simulink subsystem "S2"  (R2024b)
settings: Solver=VariableStepAuto  StartTime=0.0  StopTime=10.0  RelTol=1e-3
undefined symbols (not defined in the file): C, CC, DPL1ph, h, Half, Ll, nb_cell, numberOfCell, P_AC, Rdc, ResistanceM, Roff, Ron, Rt4, SampleTime, simetran, Ts, Zm
libraries: fl_lib x39, nesl_utility x33, ee_lib x20, simulink x6
(part 1 of 2)
Description:
  | MMC station 2
settings Model: Creator=Kyle

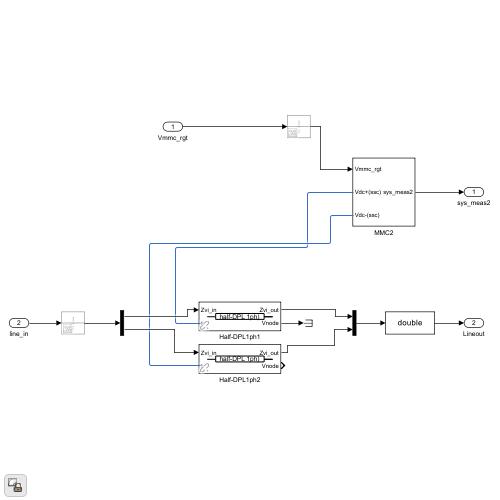
[thumbnail: Simulink's stored preview of the top-level diagram]
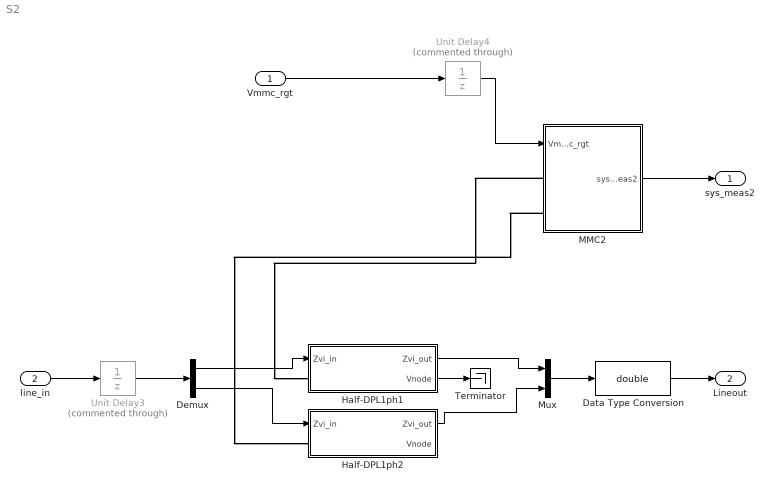
== system S2 ==
  Vmmc_rgt : Inport
  line_in : Inport  Port=2
  Data Type Conversion : DataTypeConversion  OutDataTypeStr=double  SaturateOnIntegerOverflow=off  RndMeth=Floor
  Demux : Demux  Outputs=2
  Half-DPL1ph1 : Subsystem  AncestorBlock=simetran/Half-DPL1ph  mask(Simscape 1-phase Distributed Parameters Line){Phases=1, Frequency=60, Resistance=0.015, Inductance=0.792e-3, Capacitance=14.4e-9, Length=300, Ts=Ts, cd=on}
      mask prompts: Phases "Number of phases N"; Frequency "Frequency used for R L C specification (Hz)"; Resistance "Resistance per unit length (Ohms/km)   [N*N matrix] or [R1 R0 R0m]"; Inductance "Inductance per unit length (H/km) [N*N matrix ] or [L1 L0 L0m]"; Capacitance "Capacitance per unit length (F/km) [N*N matrix] or [C1 C0 C0m]"; Length "Line length (km)"; Ts "Sample time (s)"; cd "Compensate for explicit external Unit Delay of propagation"
      mask help:
      | Implements a single-phase distributed parameter line (DPL) model.
      |
      | This DPL model allows the decoupling of computational tasks at each line ends.
      mask init:
      | % Get current block
      | currentBlock = gcb;
      | 
      | % Get electric variables
      | [Zm,R,v,Ti,to,Rt4,h,Zimp,Zmat,Yphase,ResistanceM] = ssc_dpl_cb(gcb,'variable_mask_maskinitialization', Phases, Frequency, Resistance, Inductance, Capacitance, Length);
      | % nphase=Phases;
      | % [Zm,R,v,Ti]=powericon('Distributed Parameter Line Model',nphase,Frequency,Resistance,Inductance,Capacitance);
      | %         %[Zmxx,Rmxx,Smodexx,Tixx] = blmodlin(nphase,Frequency,Resistance,Inductance,Capacitance);
      | %         %warning(w);
      | % 
      | % 
      | %         to = Length ./ v;
      | %         Rt4 = R * Length / 4;
      | %         h = (Zm - Rt4) ./ (Zm + Rt4);
      | %         Zimp = Zm + Rt4;
      | % 
      | %         % Calculate Zmat
      | %         Zmat = zeros(nphase);
      | %         for t = 1 : nphase
      | %             Zmat(t,t) = Zimp(t);
      | %         end
      | % 
      | %         % Calculate Y phase
      | %         Yphase=Ti*inv(Zmat)*(Ti');
      | % 
      | %         % Calculate R_x_0
      | %         ResistanceM = zeros(nphase);
      | %         for t = 1 : nphase
      | %             ResistanceM(t,t) = 1/(sum(Yphase(t,1:nphase)));
      | %         end
      | % 
      | %         % Calculate R_m_n
      | %         for t = 1 : nphase
      | %             for u = t+1: nphase
      | %                 ResistanceM(t,u) = -1/(Yphase(u,t));
      | %             end
      | %         end
      | V1_init=[0 zeros(1,Phases); 0.1 zeros(1,Phases)];
      | delay=floor(to/Ts);
      | if cd==1
      |     delay=delay-1;
      | end
      | if delay<1
      |     error('Line delay is less than 1 time step');
      | end
      | remd=rem(to,Ts)/Ts;
      mask TypeOptions Phases: 1 | 2 | 3 | 4 | 5 | 6 | 8 | 9 | 10 | 12
      mask Display:
      | plot(0,0,100,100,[20,20,80,80,90,80,80,20,20,10],[50,40,40,50,50,50,61,61,50,50])
      | disp('half-DPL 1ph)')
      | %disp(mess)
  Half-DPL1ph2 : Subsystem  AncestorBlock=simetran/Half-DPL1ph  mask(Simscape 1-phase Distributed Parameters Line){Phases=1, Frequency=60, Resistance=0.015, Inductance=0.792e-3, Capacitance=14.4e-9, Length=300, Ts=Ts, cd=on}
      mask prompts: Phases "Number of phases N"; Frequency "Frequency used for R L C specification (Hz)"; Resistance "Resistance per unit length (Ohms/km)   [N*N matrix] or [R1 R0 R0m]"; Inductance "Inductance per unit length (H/km) [N*N matrix ] or [L1 L0 L0m]"; Capacitance "Capacitance per unit length (F/km) [N*N matrix] or [C1 C0 C0m]"; Length "Line length (km)"; Ts "Sample time (s)"; cd "Compensate for explicit external Unit Delay of propagation"
      mask help:
      | Implements a single-phase distributed parameter line (DPL) model.
      |
      | This DPL model allows the decoupling of computational tasks at each line ends.
      mask init: same as S2/Half-DPL1ph1
      mask TypeOptions Phases: 1 | 2 | 3 | 4 | 5 | 6 | 8 | 9 | 10 | 12
      mask Display:
      | plot(0,0,100,100,[20,20,80,80,90,80,80,20,20,10],[50,40,40,50,50,50,61,61,50,50])
      | disp('half-DPL 1ph)')
      | %disp(mess)
  MMC2 : Subsystem
  Mux : Mux  Inputs=2
  Terminator : Terminator
  Unit Delay3 : UnitDelay  Commented=through  SampleTime=Ts  HasFrameUpgradeWarning=on
  Unit Delay4 : UnitDelay  Commented=through  SampleTime=Ts  HasFrameUpgradeWarning=on
  sys_meas2 : Outport
  Lineout : Outport  Port=2
  wires:
  Vmmc_rgt/1 -> Unit Delay4/1
  MMC2/1(sys_meas2) -> sys_meas2/1
  Unit Delay4/1 -> MMC2/1(Vmmc_rgt)
  Half-DPL1ph1/2(Vnode) -> Terminator/1
  Half-DPL1ph2/1(Zvi_out) -> Mux/2
  Mux/1 -> Data Type Conversion/1
  Half-DPL1ph1/1(Zvi_out) -> Mux/1
  line_in/1 -> Unit Delay3/1
  Demux/1 -> Half-DPL1ph1/1(Zvi_in)
  Demux/2 -> Half-DPL1ph2/1(Zvi_in)
  Unit Delay3/1 -> Demux/1
  Data Type Conversion/1 -> Lineout/1
  connections:
  MMC2/LConn1 -- Half-DPL1ph1/LConn1
  MMC2/LConn2 -- Half-DPL1ph2/LConn1

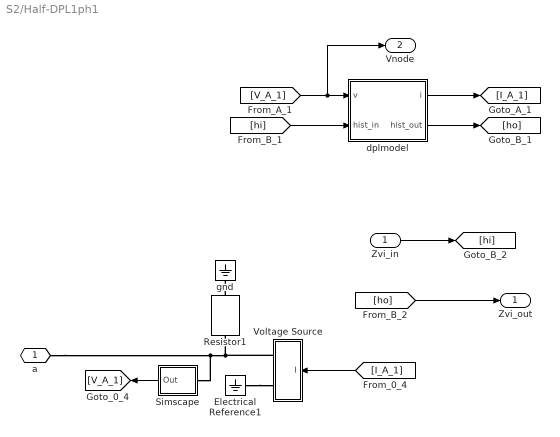
== system S2/Half-DPL1ph1 ==
  Zvi_in : Inport
  Electrical Reference1 : fl_lib/Electrical/Electrical Elements/Electrical Reference
  Resistor1 : ee_lib/Passive/Resistor  R=ResistanceM(1,1) Ohm  enable_R_tol=ee.enum.toleranceApplication.none  R_tol=5  tol_distribution=ee.enum.toleranceDistribution.uniform  nSigma=4  enable_operating_limits=ee.enum.enable.no  operating_limit_action=ee.enum.passive.reportOpLim.warn  power_rating=1 W  max_working_voltage=100 V  noise_mode=ee.enum.sources.noise.Disabled  Tdevice=25 degC  sample_time=1e-3 s  repeatability=ee.enum.ic.repeatability.notRepeatable  user_seed=0  auto_seed=3731015349  fault_action=simscape.enum.assert.action.none  t_fault=1 s  power_derating_T1=70 degC  power_derating_T2=155 degC  operating_temperature_range_vec=[-50, 150] degC  alpha=3.93e-3 1/K  Tmeas=25 degC  thermal_mass=100 J/K  temperature_specify=off  temperature_priority=High  temperature=298.15 K  temperature_nominal_specify=off  temperature_nominal_value=1  temperature_nominal_unit=K
  Simscape : Subsystem
      mask Display: disp('V')
  Voltage Source : Subsystem
  dplmodel : Subsystem
  gnd : fl_lib/Electrical/Electrical Elements/Electrical Reference
  a : PMIOPort  Side=Left
  Zvi_out : Outport  VectorParamsAs1DForOutWhenUnconnected=off
  Vnode : Outport  Port=2  VectorParamsAs1DForOutWhenUnconnected=off
  wires:
  [ho] -> Zvi_out/1
  dplmodel/1(i) -> [I_A_1]
  [V_A_1] -> Vnode/1, dplmodel/1(v)
  Zvi_in/1 -> [hi]
  [hi] -> dplmodel/2(hist_in)
  dplmodel/2(hist_out) -> [ho]
  Simscape/1(Out) -> [V_A_1]
  [I_A_1] -> Voltage Source/1(I)
  connections:
  a/RConn1 -- Simscape/LConn1 -- Voltage Source/RConn1 -- Resistor1/RConn1
  Resistor1/LConn1 -- gnd/LConn1
  Electrical Reference1/LConn1 -- Voltage Source/RConn2

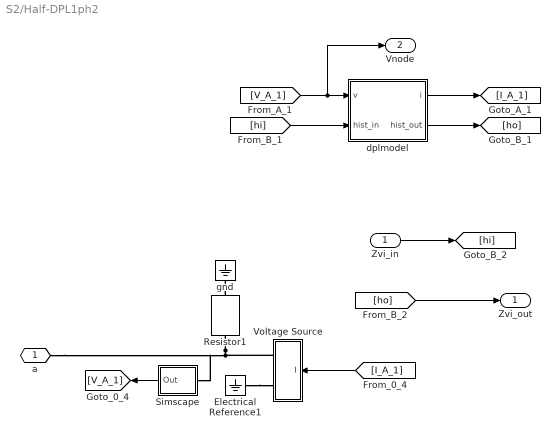
== system S2/Half-DPL1ph2 ==
  Zvi_in : Inport
  Electrical Reference1 : fl_lib/Electrical/Electrical Elements/Electrical Reference
  Resistor1 : ee_lib/Passive/Resistor  R=ResistanceM(1,1) Ohm  enable_R_tol=ee.enum.toleranceApplication.none  R_tol=5  tol_distribution=ee.enum.toleranceDistribution.uniform  nSigma=4  enable_operating_limits=ee.enum.enable.no  operating_limit_action=ee.enum.passive.reportOpLim.warn  power_rating=1 W  max_working_voltage=100 V  noise_mode=ee.enum.sources.noise.Disabled  Tdevice=25 degC  sample_time=1e-3 s  repeatability=ee.enum.ic.repeatability.notRepeatable  user_seed=0  auto_seed=362649195  fault_action=simscape.enum.assert.action.none  t_fault=1 s  power_derating_T1=70 degC  power_derating_T2=155 degC  operating_temperature_range_vec=[-50, 150] degC  alpha=3.93e-3 1/K  Tmeas=25 degC  thermal_mass=100 J/K  temperature_specify=off  temperature_priority=High  temperature=298.15 K  temperature_nominal_specify=off  temperature_nominal_value=1  temperature_nominal_unit=K
  Simscape : Subsystem
      mask Display: disp('V')
  Voltage Source : Subsystem
  dplmodel : Subsystem
  gnd : fl_lib/Electrical/Electrical Elements/Electrical Reference
  a : PMIOPort  Side=Left
  Zvi_out : Outport  VectorParamsAs1DForOutWhenUnconnected=off
  Vnode : Outport  Port=2  VectorParamsAs1DForOutWhenUnconnected=off
  wires:
  [I_A_1] -> Voltage Source/1(I)
  Simscape/1(Out) -> [V_A_1]
  dplmodel/2(hist_out) -> [ho]
  [hi] -> dplmodel/2(hist_in)
  Zvi_in/1 -> [hi]
  [V_A_1] -> dplmodel/1(v), Vnode/1
  dplmodel/1(i) -> [I_A_1]
  [ho] -> Zvi_out/1
  connections:
  Electrical Reference1/LConn1 -- Voltage Source/RConn2
  Resistor1/LConn1 -- gnd/LConn1
  Resistor1/RConn1 -- Voltage Source/RConn1 -- Simscape/LConn1 -- a/RConn1

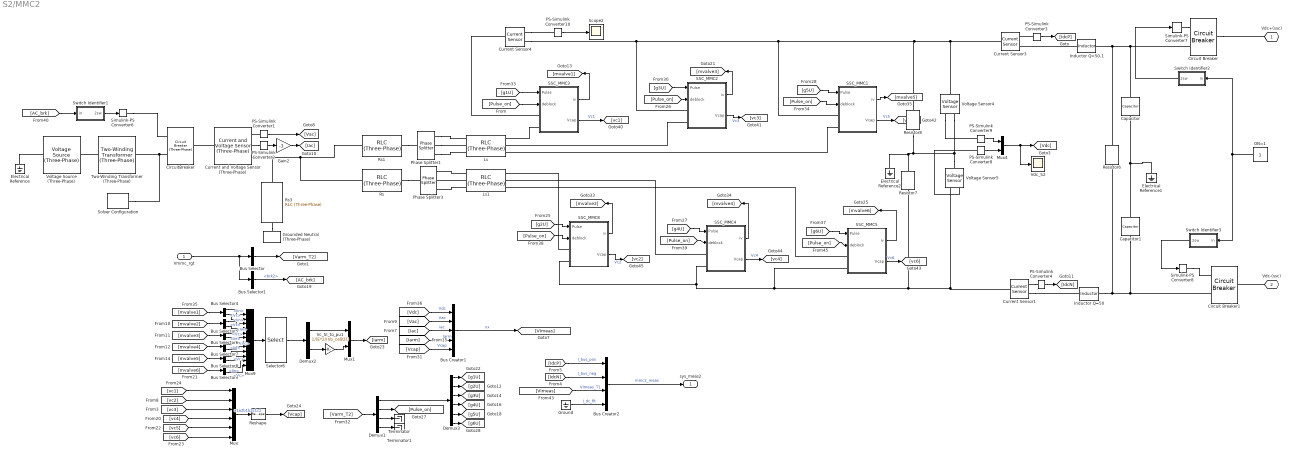
== system S2/MMC2 ==
  Vmmc_rgt : Inport
  " Switch Identifier1" : Subsystem  mask{bn=brk1, bns=brk1, rsw=on}
      mask prompts: bn "Switch block name (no ' ')"; bns "saved blockname"; rsw "Reverse switch logic"
      mask DialogControl Control2 Prompt: Note: Simscape electric breaker in open (OFF) when gate=1)
      mask DialogControl Control3 Prompt: Note: by using revert logic, it becomes like SPS breaker
  " Switch Identifier2" : Subsystem  mask{bn=brk1, bns=brk1, rsw=on}
      mask prompts: bn "Switch block name (no ' ')"; bns "saved blockname"; rsw "Reverse switch logic"
      mask DialogControl Control2 Prompt: Note: Simscape electric breaker in open (OFF) when gate=1)
      mask DialogControl Control3 Prompt: Note: by using revert logic, it becomes like SPS breaker
  " Switch Identifier3" : Subsystem  mask{bn=brk1, bns=brk1, rsw=on}
      mask prompts: bn "Switch block name (no ' ')"; bns "saved blockname"; rsw "Reverse switch logic"
      mask DialogControl Control2 Prompt: Note: Simscape electric breaker in open (OFF) when gate=1)
      mask DialogControl Control3 Prompt: Note: by using revert logic, it becomes like SPS breaker
  Bus Creator1 : BusCreator  Inputs=5
  Bus Creator2 : BusCreator  Inputs=4  OutDataTypeStr=Bus: mmc2_meas  NonVirtualBus=on
  Bus Selector : BusSelector  OutputSignals=pulse,dblk_rgt,para  OutputAsBus=on
  Bus Selector1 : BusSelector  OutputSignals=brk2
  Bus Selector{4..9} (6 alike) : BusSelector  OutputSignals=Iin,Vc
  Capacitor : ee_lib/Passive/Capacitor  cap_option=ee.enum.passive.capacitor.capOption.const  c=2.5e-6 F  Cvec=[1e-05, 1e-06] F  Vvec=[0, 10] V  CV_table_symmetry=ee.enum.passive.capacitor.tableSymmetry.yes  f_vec=[1, 10] kHz  DFext_vec=[.8, 1.2]  enable_C_tol=ee.enum.toleranceApplication.none  averaging_period=0 s  C_tol=5  tol_distribution=ee.enum.toleranceDistribution.uniform  nSigma=4  r=0 Ohm  g=0 1/Ohm  enable_operating_limits=ee.enum.enable.no  operating_limit_action=ee.enum.passive.reportOpLim.warn  max_working_voltage_range=[-25, 25] V  power_rating=1 W  maxTemperature=85 degC  thermalEnable=false  thermalMass=1 J/K  fault_action=simscape.enum.assert.action.none  t_fault=1 s  i_specify=off  i_priority=None  i=0 A  i_nominal_specify=off  i_nominal_value=1  i_nominal_unit=A  v_specify=off  v_priority=None  v=0 V  v_nominal_specify=off  v_nominal_value=1  v_nominal_unit=V  vc_specify=off  vc_priority=High  vc=0 V  vc_nominal_specify=off  vc_nominal_value=1  vc_nominal_unit=V  T_specify=off  T_priority=None  T=298.15 K  T_nominal_specify=off  T_nominal_value=1  T_nominal_unit=K
  Capacitor1 : ee_lib/Passive/Capacitor  cap_option=ee.enum.passive.capacitor.capOption.const  c=2.5e-6 F  Cvec=[1e-05, 1e-06] F  Vvec=[0, 10] V  CV_table_symmetry=ee.enum.passive.capacitor.tableSymmetry.yes  f_vec=[1, 10] kHz  DFext_vec=[.8, 1.2]  enable_C_tol=ee.enum.toleranceApplication.none  averaging_period=0 s  C_tol=5  tol_distribution=ee.enum.toleranceDistribution.uniform  nSigma=4  r=0 Ohm  g=0 1/Ohm  enable_operating_limits=ee.enum.enable.no  operating_limit_action=ee.enum.passive.reportOpLim.warn  max_working_voltage_range=[-25, 25] V  power_rating=1 W  maxTemperature=85 degC  thermalEnable=false  thermalMass=1 J/K  fault_action=simscape.enum.assert.action.none  t_fault=1 s  i_specify=off  i_priority=None  i=0 A  i_nominal_specify=off  i_nominal_value=1  i_nominal_unit=A  v_specify=off  v_priority=None  v=0 V  v_nominal_specify=off  v_nominal_value=1  v_nominal_unit=V  vc_specify=off  vc_priority=High  vc=0 V  vc_nominal_specify=off  vc_nominal_value=1  vc_nominal_unit=V  T_specify=off  T_priority=None  T=298.15 K  T_nominal_specify=off  T_nominal_value=1  T_nominal_unit=K
  Circuit Breaker : ee_lib/Switches & Breakers/Circuit Breaker  R_closed=0.001 Ohm  G_open=1e-6 1/Ohm  threshold=0.5 V  breaker_behavior=ee.enum.switches.breakerBehavior.zeroCrossingEnable
      settings: InternalSimscapePortConfiguration="{\"Bottom\":[],\"Left\":[{\"id\":\"vT\",\"label\":\"vT\",\"type\":\"input\"},{\"id\":\"p1\",\"label\":\"\",\"type\":\"foundation.electrical.electrical\"}],\"Right\":[{\"id\":\"p2\",\"label\":\"\",\"type\":\"foundation.electrical.electrical\"}],\"Top\":[]}"
  Circuit Breaker1 : ee_lib/Switches & Breakers/Circuit Breaker  R_closed=0.001 Ohm  G_open=1e-6 1/Ohm  threshold=0.5 V  breaker_behavior=ee.enum.switches.breakerBehavior.zeroCrossingEnable
      settings: InternalSimscapePortConfiguration="{\"Bottom\":[],\"Left\":[{\"id\":\"vT\",\"label\":\"vT\",\"type\":\"input\"},{\"id\":\"p1\",\"label\":\"\",\"type\":\"foundation.electrical.electrical\"}],\"Right\":[{\"id\":\"p2\",\"label\":\"\",\"type\":\"foundation.electrical.electrical\"}],\"Top\":[]}"
  CircuitBreaker : ee_lib/Switches & Breakers/Circuit Breaker (Three-Phase)  R_closed=0.001 Ohm  G_open=1/1000 1/Ohm  threshold=0.5 V  breaker_behavior=ee.enum.switches.breakerBehavior.zeroCrossingEnable
      settings: InternalSimscapePortConfiguration="{\"Bottom\":[],\"Left\":[{\"id\":\"vT\",\"label\":\"vT\",\"type\":\"input\"},{\"id\":\"N1\",\"label\":\"~1\",\"type\":\"foundation.electrical.three_phase\"}],\"Right\":[{\"id\":\"N2\",\"label\":\"~2\",\"type\":\"foundation.electrical.three_phase\"}],\"Top\":[]}"
  Current Sensor1 : fl_lib/Electrical/Electrical Sensors/Current Sensor
  Current Sensor3 : fl_lib/Electrical/Electrical Sensors/Current Sensor
  Current Sensor4 : fl_lib/Electrical/Electrical Sensors/Current Sensor
  Current and Voltage Sensor (Three-Phase) : ee_lib/Sensors & Transducers/Current and Voltage Sensor (Three-Phase)  vMeasurementType=ee.enum.vmeasurement.lg  outputUnit=ee.enum.unit.si  SRated=100e6 A*V  VRated=24e3 V  I_specify=off  I_priority=None  I=[0, 0, 0] A  I_nominal_specify=off  I_nominal_value=1  I_nominal_unit=A  V_specify=off  V_priority=None  V=[0, 0, 0] V  V_nominal_specify=off  V_nominal_value=1  V_nominal_unit=V
      settings: InternalSimscapePortConfiguration="{\"Bottom\":[],\"Left\":[{\"id\":\"N1\",\"label\":\"~1\",\"type\":\"foundation.electrical.three_phase\"}],\"Right\":[{\"id\":\"V_output\",\"label\":\"V\",\"type\":\"output\"},{\"id\":\"I_output\",\"label\":\"I\",\"type\":\"output\"},{\"id\":\"N2\",\"label\":\"~2\",\"type\":\"foundation.electrical.three_phase\"}],\"Top\":[]}"
  Demux1 : Demux  Outputs=[numberOfCell*6 1 5 1]
  Demux2 : Demux  Outputs=[6 6]
  Demux3 : Demux  Outputs=ones(6,1)*numberOfCell
  Electrical Reference : fl_lib/Electrical/Electrical Elements/Electrical Reference
  Electrical Reference1 : fl_lib/Electrical/Electrical Elements/Electrical Reference
  Electrical Reference2 : fl_lib/Electrical/Electrical Elements/Electrical Reference
  Gain2 : Gain  Gain=-1
  Ground : Ground
  Grounded Neutral (Three-Phase) : ee_lib/Connectors & References/Grounded Neutral (Three-Phase)
  Inductor Q=50 : ee_lib/Passive/Inductor  l=10e-3 H  enable_L_tol=ee.enum.toleranceApplication.none  L_tol=20  tol_distribution=ee.enum.toleranceDistribution.uniform  nSigma=4  r=2*pi*50/50*10e-3 Ohm  g=1e-9 1/Ohm  enable_operating_limits=ee.enum.enable.no  operating_limit_action=ee.enum.passive.reportOpLim.warn  max_working_current=1 A  power_rating=1 W  fault_action=simscape.enum.assert.action.none  t_fault=1 s  i_L_specify=off  i_L_priority=High  i_L=0 A  i_L_nominal_specify=off  i_L_nominal_value=1  i_L_nominal_unit=A
  Inductor Q=50.1 : ee_lib/Passive/Inductor  l=10e-3 H  enable_L_tol=ee.enum.toleranceApplication.none  L_tol=20  tol_distribution=ee.enum.toleranceDistribution.uniform  nSigma=4  r=2*pi*50/50*10e-3 Ohm  g=1e-9 1/Ohm  enable_operating_limits=ee.enum.enable.no  operating_limit_action=ee.enum.passive.reportOpLim.warn  max_working_current=1 A  power_rating=1 W  fault_action=simscape.enum.assert.action.none  t_fault=1 s  i_L_specify=off  i_L_priority=High  i_L=0 A  i_L_nominal_specify=off  i_L_nominal_value=1  i_L_nominal_unit=A
  Ls : ee_lib/Passive/RLC Assemblies/RLC (Three-Phase)  port_option=ee.enum.threePhasePort.expanded  component_structure=ee.enum.rlc.structure.ParallelRL  R=Ll*2*pi*10000 Ohm  L=Ll H  C=1e-6 F  R_parasitic=0 Ohm  G_parasitic=0 1/Ohm  IL_specify=off  IL_priority=High  IL=[0, 0, 0] A  IL_nominal_specify=off  IL_nominal_value=1  IL_nominal_unit=A  VC_specify=off  VC_priority=High  VC=[0, 0, 0] V  VC_nominal_specify=off  VC_nominal_value=1  VC_nominal_unit=V
      settings: InternalSimscapePortConfiguration="{\"Bottom\":[],\"Left\":[{\"id\":\"a1\",\"label\":\"a1\",\"type\":\"foundation.electrical.electrical\"},{\"id\":\"b1\",\"label\":\"b1\",\"type\":\"foundation.electrical.electrical\"},{\"id\":\"c1\",\"label\":\"c1\",\"type\":\"foundation.electrical.electrical\"}],\"Right\":[{\"id\":\"a2\",\"label\":\"a2\",\"type\":\"foundation.electrical.electrical\"},{\"id\":\"b2\",\"label\":\"b2\",\"type\":\"foundation.electrical.electrical\"},{\"id\":\"c2\",\"label\":\"c2\",\"type\":\"foundation.electrical.electrical\"}],\"Top\":[]}"
  Ls1 : ee_lib/Passive/RLC Assemblies/RLC (Three-Phase)  port_option=ee.enum.threePhasePort.expanded  component_structure=ee.enum.rlc.structure.ParallelRL  R=Ll*2*pi*10000 Ohm  L=Ll H  C=1e-6 F  R_parasitic=0 Ohm  G_parasitic=0 1/Ohm  IL_specify=off  IL_priority=High  IL=[0, 0, 0] A  IL_nominal_specify=off  IL_nominal_value=1  IL_nominal_unit=A  VC_specify=off  VC_priority=High  VC=[0, 0, 0] V  VC_nominal_specify=off  VC_nominal_value=1  VC_nominal_unit=V
      settings: InternalSimscapePortConfiguration="{\"Bottom\":[],\"Left\":[{\"id\":\"a1\",\"label\":\"a1\",\"type\":\"foundation.electrical.electrical\"},{\"id\":\"b1\",\"label\":\"b1\",\"type\":\"foundation.electrical.electrical\"},{\"id\":\"c1\",\"label\":\"c1\",\"type\":\"foundation.electrical.electrical\"}],\"Right\":[{\"id\":\"a2\",\"label\":\"a2\",\"type\":\"foundation.electrical.electrical\"},{\"id\":\"b2\",\"label\":\"b2\",\"type\":\"foundation.electrical.electrical\"},{\"id\":\"c2\",\"label\":\"c2\",\"type\":\"foundation.electrical.electrical\"}],\"Top\":[]}"
  Mux : Mux  Inputs=ones(6,1)*numberOfCell
  Mux1 : Mux  Inputs=2
  Mux4 : Mux  Inputs=2
  Mux9 : Mux  Inputs=12
  ON=1 : Constant
  PS-Simulink Converter{1..4,8..10} (7 alike) : nesl_utility/PS-Simulink Converter  PhysicalDomain=network_engine_domain  SubClassName=ps_output  LeftPortType=input  RightPortType=output  PseudoPeriodic=off  Frequencies=[]  VectorFormat=inherit  Unit=inherit  AffineConversion=off
  Phase Splitter1 : ee_lib/Connectors & References/Phase Splitter
  Phase Splitter3 : ee_lib/Connectors & References/Phase Splitter
  Reshape : Reshape
  Resistor6 : fl_lib/Electrical/Electrical Elements/Resistor  R=1000000 Ohm  i_specify=off  i_priority=None  i=0 A  i_nominal_specify=off  i_nominal_value=1  i_nominal_unit=A  v_specify=off  v_priority=None  v=0 V  v_nominal_specify=off  v_nominal_value=1  v_nominal_unit=V
  Resistor7 : fl_lib/Electrical/Electrical Elements/Resistor  R=Rdc Ohm  i_specify=off  i_priority=None  i=0 A  i_nominal_specify=off  i_nominal_value=1  i_nominal_unit=A  v_specify=off  v_priority=None  v=0 V  v_nominal_specify=off  v_nominal_value=1  v_nominal_unit=V
  Resistor8 : fl_lib/Electrical/Electrical Elements/Resistor  R=Rdc Ohm  i_specify=off  i_priority=None  i=0 A  i_nominal_specify=off  i_nominal_value=1  i_nominal_unit=A  v_specify=off  v_priority=None  v=0 V  v_nominal_specify=off  v_nominal_value=1  v_nominal_unit=V
  Rs : ee_lib/Passive/RLC Assemblies/RLC (Three-Phase)  port_option=ee.enum.threePhasePort.composite  component_structure=ee.enum.rlc.structure.R  R=0.0001 Ohm  L=Ll H  C=1e-6 F  R_parasitic=0 Ohm  G_parasitic=0 1/Ohm  IL_specify=off  IL_priority=High  IL=[0, 0, 0] A  IL_nominal_specify=off  IL_nominal_value=1  IL_nominal_unit=A  VC_specify=off  VC_priority=High  VC=[0, 0, 0] V  VC_nominal_specify=off  VC_nominal_value=1  VC_nominal_unit=V
      settings: InternalSimscapePortConfiguration="{\"Bottom\":[],\"Left\":[{\"id\":\"N1\",\"label\":\"~1\",\"type\":\"foundation.electrical.three_phase\"}],\"Right\":[{\"id\":\"N2\",\"label\":\"~2\",\"type\":\"foundation.electrical.three_phase\"}],\"Top\":[]}"
  Rs1 : ee_lib/Passive/RLC Assemblies/RLC (Three-Phase)  port_option=ee.enum.threePhasePort.composite  component_structure=ee.enum.rlc.structure.R  R=0.0001 Ohm  L=Ll H  C=1e-6 F  R_parasitic=0 Ohm  G_parasitic=0 1/Ohm  IL_specify=off  IL_priority=High  IL=[0, 0, 0] A  IL_nominal_specify=off  IL_nominal_value=1  IL_nominal_unit=A  VC_specify=off  VC_priority=High  VC=[0, 0, 0] V  VC_nominal_specify=off  VC_nominal_value=1  VC_nominal_unit=V
      settings: InternalSimscapePortConfiguration="{\"Bottom\":[],\"Left\":[{\"id\":\"N1\",\"label\":\"~1\",\"type\":\"foundation.electrical.three_phase\"}],\"Right\":[{\"id\":\"N2\",\"label\":\"~2\",\"type\":\"foundation.electrical.three_phase\"}],\"Top\":[]}"
  Rs3 : ee_lib/Passive/RLC Assemblies/RLC (Three-Phase)  port_option=ee.enum.threePhasePort.composite  component_structure=ee.enum.rlc.structure.R  R=1e6 Ohm  L=Ll H  C=1e-6 F  R_parasitic=0 Ohm  G_parasitic=0 1/Ohm  IL_specify=off  IL_priority=High  IL=[0, 0, 0] A  IL_nominal_specify=off  IL_nominal_value=1  IL_nominal_unit=A  VC_specify=off  VC_priority=High  VC=[0, 0, 0] V  VC_nominal_specify=off  VC_nominal_value=1  VC_nominal_unit=V
      settings: InternalSimscapePortConfiguration="{\"Bottom\":[],\"Left\":[{\"id\":\"N1\",\"label\":\"~1\",\"type\":\"foundation.electrical.three_phase\"}],\"Right\":[{\"id\":\"N2\",\"label\":\"~2\",\"type\":\"foundation.electrical.three_phase\"}],\"Top\":[]}"
  SSC_MMC1 : Subsystem  mask(SimScape MMC module (half-bridge)){nbc=200, ron=Ron, roff=Roff, cc=CC, Ts=Ts, rf=on, dts=on}
      mask prompts: nbc "Number of cell"; ron "IGBT Ron (Ohms)"; roff "IGBT Roff (Ohms)"; cc "Cell capacitance (F)"; Ts "Sample Time (s)"; rf "Non-infinite Roff"; dts "Disabled time stamping"
      mask help: This model implements an half-bridge MMC module with full nodal solution, i.e. there is no delay between the MMC and then main solver solution and the MMC module is seen as a discrete Thevenin equivalent to the main Simscape solver.
      mask init:
      | for k=1:4
      |     switch k
      |          case 1
      |               R1=roff; R2=roff;
      |               A(k)=0; B(k)=0; C(k)=0; D(k)=R2;
      |          case 2
      |               R1=ron; R2=roff;
      |               A(k)=0; B(k)=1/cc; C(k)=1; D(k)=R1;
      |          case 3
      |               R1=roff; R2=ron;
      |               A(k)=0; B(k)=0; C(k)=0; D(k)=R2;
      |          case 4
      |              R1=ron; R2=ron;
      |              A(k)=0; B(k)=0; C(k)=0; D(k)=R2; %incorrect but not supposed to happen
      |     end
      |     if isequal(get_param(gcb,'rf'),'on')
      |      rr=(1+R2/R1);
      |      A(k)=-1/R1/cc/rr;
      |      B(k)=R2/R1/cc/rr;
      |      C(k)=R2/R1/rr;
      |      D(k)=R2/rr;
      |     end
      |          
      |        %% choose here if you want trapeze or backward Euler (more stable) 
      |         if 1==0 % trap
      |             Ad(k) = (1-Ts/2*A(k))\(1+Ts/2*A(k));         %SS discretize
      |             Bd1(k) = (1-Ts/2*A(k))\(Ts/2*B(k));    %SS discretize
      |             Bd2(k) = (1-Ts/2*A(k))\(Ts/2*B(k));    %SS discretize
      |         else % BE
      |             Ad(k) = 1/(1-Ts*A(k));         %SS discretize
      |             Bd2(k) = Ts*B(k)/(1-Ts*A(k));    %SS discretize
      |             Bd1(k) =0;
      |         end
      |         Z(k)=C(k)'.*Bd2(k) + D(k);
      | end
      | 
      | 
      | dtsval=1; %must be = 1
      mask Display: disp('MMC arm')
  SSC_MMC2 : Subsystem  mask(SimScape MMC module (half-bridge)){nbc=200, ron=Ron, roff=Roff, cc=CC, Ts=Ts, rf=on, dts=on}
      mask prompts: nbc "Number of cell"; ron "IGBT Ron (Ohms)"; roff "IGBT Roff (Ohms)"; cc "Cell capacitance (F)"; Ts "Sample Time (s)"; rf "Non-infinite Roff"; dts "Disabled time stamping"
      mask help: This model implements an half-bridge MMC module with full nodal solution, i.e. there is no delay between the MMC and then main solver solution and the MMC module is seen as a discrete Thevenin equivalent to the main Simscape solver.
      mask init: same as S2/MMC2/SSC_MMC1
      mask Display: disp('MMC arm')
  SSC_MMC3 : Subsystem  mask(SimScape MMC module (half-bridge)){nbc=200, ron=Ron, roff=Roff, cc=CC, Ts=Ts, rf=on, dts=on}
      mask prompts: nbc "Number of cell"; ron "IGBT Ron (Ohms)"; roff "IGBT Roff (Ohms)"; cc "Cell capacitance (F)"; Ts "Sample Time (s)"; rf "Non-infinite Roff"; dts "Disabled time stamping"
      mask help: This model implements an half-bridge MMC module with full nodal solution, i.e. there is no delay between the MMC and then main solver solution and the MMC module is seen as a discrete Thevenin equivalent to the main Simscape solver.
      mask init: same as S2/MMC2/SSC_MMC1
      mask Display: disp('MMC arm')
  SSC_MMC4 : Subsystem  mask(SimScape MMC module (half-bridge)){nbc=200, ron=Ron, roff=Roff, cc=CC, Ts=Ts, rf=on, dts=on}
      mask prompts: nbc "Number of cell"; ron "IGBT Ron (Ohms)"; roff "IGBT Roff (Ohms)"; cc "Cell capacitance (F)"; Ts "Sample Time (s)"; rf "Non-infinite Roff"; dts "Disabled time stamping"
      mask help: This model implements an half-bridge MMC module with full nodal solution, i.e. there is no delay between the MMC and then main solver solution and the MMC module is seen as a discrete Thevenin equivalent to the main Simscape solver.
      mask init: same as S2/MMC2/SSC_MMC1
      mask Display: disp('MMC arm')
  SSC_MMC5 : Subsystem  mask(SimScape MMC module (half-bridge)){nbc=200, ron=Ron, roff=Roff, cc=CC, Ts=Ts, rf=on, dts=on}
      mask prompts: nbc "Number of cell"; ron "IGBT Ron (Ohms)"; roff "IGBT Roff (Ohms)"; cc "Cell capacitance (F)"; Ts "Sample Time (s)"; rf "Non-infinite Roff"; dts "Disabled time stamping"
      mask help: This model implements an half-bridge MMC module with full nodal solution, i.e. there is no delay between the MMC and then main solver solution and the MMC module is seen as a discrete Thevenin equivalent to the main Simscape solver.
      mask init: same as S2/MMC2/SSC_MMC1
      mask Display: disp('MMC arm')
  SSC_MMC8 : Subsystem  mask(SimScape MMC module (half-bridge)){nbc=200, ron=Ron, roff=Roff, cc=CC, Ts=Ts, rf=on, dts=on}
      mask prompts: nbc "Number of cell"; ron "IGBT Ron (Ohms)"; roff "IGBT Roff (Ohms)"; cc "Cell capacitance (F)"; Ts "Sample Time (s)"; rf "Non-infinite Roff"; dts "Disabled time stamping"
      mask help: This model implements an half-bridge MMC module with full nodal solution, i.e. there is no delay between the MMC and then main solver solution and the MMC module is seen as a discrete Thevenin equivalent to the main Simscape solver.
      mask init: same as S2/MMC2/SSC_MMC1
      mask Display: disp('MMC arm')
  Scope2 : Scope
  Selector6 : Selector  InputPortWidth=12  IndexOptions=Index vector (dialog)  Indices=[1:2:12,2:2:12]  OutputSizes=1
  Simulink-PS Converter6 : nesl_utility/Simulink-PS Converter  PhysicalDomain=network_engine_domain  SubClassName=ps_input  LeftPortType=input  RightPortType=output  PseudoPeriodic=off  Frequencies=[]  NoiseDistribution=none  NoiseParameters=[]  Unit=1  AffineConversion=off  FilteringAndDerivatives=provide  SimscapeFilterOrder=1  InputFilterTimeConstant=0.001  UdotUserProvided=0
  Simulink-PS Converter7 : nesl_utility/Simulink-PS Converter  PhysicalDomain=network_engine_domain  SubClassName=ps_input  LeftPortType=input  RightPortType=output  PseudoPeriodic=off  Frequencies=[]  NoiseDistribution=none  NoiseParameters=[]  Unit=1  AffineConversion=off  FilteringAndDerivatives=provide  SimscapeFilterOrder=1  InputFilterTimeConstant=0.001  UdotUserProvided=0
  Simulink-PS Converter8 : nesl_utility/Simulink-PS Converter  PhysicalDomain=network_engine_domain  SubClassName=ps_input  LeftPortType=input  RightPortType=output  PseudoPeriodic=off  Frequencies=[]  NoiseDistribution=none  NoiseParameters=[]  Unit=1  AffineConversion=off  FilteringAndDerivatives=provide  SimscapeFilterOrder=1  InputFilterTimeConstant=0.001  UdotUserProvided=0
  Solver Configuration : nesl_utility/Solver Configuration  PhysicalDomain=network_engine_domain  SubClassName=solver  LeftPortType=input  RightPortType=generic  Tones=[]  Harmonics=[]  SimulateNoise=off  Profile=off  UseLocalSampling=off  EnableSwitchedLinearOptims=on  FrequencyDomain=off  UseCCode=off  RelTol=0.001  AbsTol=0.001  MinStep=1e-09  ToWorkspace=off  RevertToSquareIcSolve=off  NumHomotopyIterations=100  PhasorMode=off  PhasorModeNumHarmonics=1  ConsistencySolver=NEWTON_XTOL_AFTER_FTOL  IndexReductionMethod=None  DoDC=off  ResidualTolerance=1e-09  ConsistencyTolSource=GLOBAL  ConsistencyAbsTol=0.001  ConsistencyRelTol=0.001  ConsistencyTolFactor=0.001  UseLocalSolver=on  LocalSolverChoice=NE_TRAPEZOIDAL_ADVANCER  ResolveIndetEquations=off  FunctionEvalNumThread=1  LocalSolverSampleTime=Ts  DoFixedCost=on  MaxNonlinIter=1  MaxModeIter=2  ComputeImpulses=off  ImpulseIterations=2  LinearAlgebra=auto  LinearAlgebraNumThread=0  EquationFormulation=NE_TIME_EF  DelaysMemoryBudget=1024  AutomaticFiltering=off  FilteringTimeConstant=0.001  PartitionStorageMethod=AS_NEEDED  PartitionMemoryBudget=1024  PartitionMethod=ROBUST  MultibodyUseLocalSolver=off  MultibodyLocalSolverChoice=ODE1  MultibodyLocalSolverSampleTime=0.001
  Terminator : Terminator
  Terminator1 : Terminator
  Two-Winding Transformer (Three-Phase) : ee_lib/Passive/Transformers/Two-Winding Transformer (Three-Phase)  SRated=S_Xfo A*V  FRated=freq_right Hz  Winding1Connection=ee.enum.windingconnection.Yg  VRated1="V_AC_prim   V"  Winding2Connection=ee.enum.windingconnection.Y  VRated2=V_AC_sec V  CoreType=ee.enum.coretype.fivelimb  pu_Rw1=0.0025  pu_Rw2=0.0025  leakage_reactance_option=ee.enum.transformer_leakage.include  pu_Xl1=0.05  pu_Xl2=0.05  magnetizing_resistance_option=ee.enum.transformer_magnetizingResistance.include  pu_Rm=167  magnetizing_reactance_option=ee.enum.transformer_magnetizingReactance.include  saturation_option=ee.enum.transformer_saturation.exclude  pu_Xm=167  current_data=[0, .002, 1, 2]  magnetic_flux_data=[0, 1.2, 1.5, 1.51]  pu_X0=0.5  i1_specify=off  i1_priority=None  i1=[0, 0, 0] A  i1_nominal_specify=off  i1_nominal_value=1  i1_nominal_unit=A  i2_specify=off  i2_priority=None  i2=[0, 0, 0] A  i2_nominal_specify=off  i2_nominal_value=1  i2_nominal_unit=A  phi_specify=off  phi_priority=None  phi=[0, 0, 0]  phi_nominal_specify=off  phi_nominal_value=1  phi_nominal_unit=1  power_dissipated_specify=off  power_dissipated_priority=None  power_dissipated=0 W  power_dissipated_nominal_specify=off  power_dissipated_nominal_value=1  power_dissipated_nominal_unit=W
      settings: InternalSimscapePortConfiguration="{\"Bottom\":[],\"Left\":[{\"id\":\"N1\",\"label\":\"~1\",\"type\":\"foundation.electrical.three_phase\"}],\"Right\":[{\"id\":\"N2\",\"label\":\"~2\",\"type\":\"foundation.electrical.three_phase\"}],\"Top\":[]}"
  Vc_SI_to_pu1 : Gain  Gain=1/(E*2/(nb_cell/2))  SampleTime=Ts
  Vdc_S2 : Scope
  Voltage Source (Three-Phase) : ee_lib/Sources/Voltage Source (Three-Phase)  vline_rms=V_AC_prim V  shift=0 deg  freq=freq_right Hz  impedance_option=1  SShortCircuit=P_AC*20 A*V  XR=20  R=0.01 Ohm  L=3.97e-4 H  harmonic_option=0  harmonic_orders=[5, 7, 11, 13]  harmonic_ratios=[.1, .1, .1, .1]  G_parasitic=0 1/Ohm  I_specify=off  I_priority=None  I=[0, 0, 0] A  I_nominal_specify=off  I_nominal_value=1  I_nominal_unit=A
  Voltage Sensor4 : fl_lib/Electrical/Electrical Sensors/Voltage Sensor
  Voltage Sensor5 : fl_lib/Electrical/Electrical Sensors/Voltage Sensor
  Vdc+(ssc) : PMIOPort  Tag=PMCPort  Side=Left
  Vdc-(ssc) : PMIOPort  Tag=PMCPort  Port=2  Side=Left
  sys_meas2 : Outport  VectorParamsAs1DForOutWhenUnconnected=off
  wires:
  [g3U] -> SSC_MMC2/1(Pulse)
  [g1U] -> SSC_MMC3/1(Pulse)
  [Pulse_on] -> SSC_MMC3/2(deblock)
  ON=1/1 -> " Switch Identifier3"/1(in), " Switch Identifier2"/1(in)
  PS-Simulink Converter9/1 -> Mux4/1
  SSC_MMC5/2(Vcap) -> [vc6]  "Vc6"
  SSC_MMC5/1(iv) -> [mvalve6]
  SSC_MMC8/2(Vcap) -> [vc2]  "Vc2"
  SSC_MMC8/1(iv) -> [mvalve2]
  PS-Simulink Converter10/1 -> Scope2/1
  PS-Simulink Converter8/1 -> Mux4/2
  Mux4/1 -> Vdc_S2/1, [Vdc]
  SSC_MMC1/2(Vcap) -> [vc5]  "Vc5"
  PS-Simulink Converter3/1 -> [IdcP]
  [Pulse_on] -> SSC_MMC5/2(deblock)
  PS-Simulink Converter4/1 -> [IdcN]
  [Pulse_on] -> SSC_MMC8/2(deblock)
  SSC_MMC3/2(Vcap) -> [vc1]  "Vc1"
  SSC_MMC4/2(Vcap) -> [vc4]  "Vc4"
  SSC_MMC4/1(iv) -> [mvalve4]
  [Pulse_on] -> SSC_MMC4/2(deblock)
  [Pulse_on] -> SSC_MMC1/2(deblock)
  [g5U] -> SSC_MMC1/1(Pulse)
  SSC_MMC3/1(iv) -> [mvalve1]
  SSC_MMC1/1(iv) -> [mvalve5]
  [g4U] -> SSC_MMC4/1(Pulse)
  [g2U] -> SSC_MMC8/1(Pulse)
  [g6U] -> SSC_MMC5/1(Pulse)
  [Pulse_on] -> SSC_MMC2/2(deblock)
  SSC_MMC2/1(iv) -> [mvalve3]
  SSC_MMC2/2(Vcap) -> [vc3]  "Vc3"
  [Iac] -> Bus Creator1/3  "Iac"
  PS-Simulink Converter1/1 -> [Vac]
  Bus Creator2/1 -> sys_meas2/1  "mmc2_meas"
  [VImeas] -> Bus Creator2/3  "VImeas_T1"
  Demux2/1 -> Mux1/1
  Gain2/1 -> [Iac]
  [vc2] -> Mux/2
  Demux1/3 -> Terminator/1
  Mux9/1 -> Selector6/1
  Bus Selector4/2 -> Mux9/2  "<Vc>"
  [Varm_T2] -> Demux1/1
  [Vac] -> Bus Creator1/2  "Vac"
  [AC_brk] -> " Switch Identifier1"/1(in)
  Demux3/1 -> [g1U]
  Bus Creator1/1 -> [VImeas]  "xx"
  Demux3/6 -> [g6U]
  [mvalve1] -> Bus Selector4/1
  Mux/1 -> Reshape/1  "a1a2b1b2c1c2"
  Bus Selector9/1 -> Mux9/11  "<Iin>"
  [vc3] -> Mux/3
  [vc1] -> Mux/1
  Bus Selector4/1 -> Mux9/1  "<Iin>"
  [Iarm] -> Bus Creator1/4  "Iarm"
  Vc_SI_to_pu1/1 -> Mux1/2
  [Vdc] -> Bus Creator1/1  "Vdc"
  Demux1/2 -> [Pulse_on]
  Demux1/4 -> Terminator1/1
  PS-Simulink Converter2/1 -> Gain2/1
  Demux3/5 -> [g5U]
  [mvalve4] -> Bus Selector7/1
  Mux1/1 -> [Iarm]
  Demux1/1 -> Demux3/1
  [vc4] -> Mux/4
  Demux3/3 -> [g3U]
  [mvalve6] -> Bus Selector9/1
  Selector6/1 -> Demux2/1
  Ground/1 -> Bus Creator2/4  "I_dc_flt"
  [vc5] -> Mux/5
  [Vcap] -> Bus Creator1/5  "Vcap"
  Demux3/2 -> [g2U]
  [vc6] -> Mux/6
  Demux3/4 -> [g4U]
  Demux2/2 -> Vc_SI_to_pu1/1
  [IdcP] -> Bus Creator2/1  "I_bus_pos"
  [mvalve5] -> Bus Selector8/1
  [mvalve2] -> Bus Selector5/1
  [IdcN] -> Bus Creator2/2  "I_bus_neg"
  [mvalve3] -> Bus Selector6/1
  Bus Selector8/1 -> Mux9/9  "<Iin>"
  Reshape/1 -> [Vcap]
  Bus Selector9/2 -> Mux9/12  "<Vc>"
  Bus Selector6/2 -> Mux9/6  "<Vc>"
  Bus Selector5/2 -> Mux9/4  "<Vc>"
  Bus Selector5/1 -> Mux9/3  "<Iin>"
  Bus Selector7/2 -> Mux9/8  "<Vc>"
  Bus Selector7/1 -> Mux9/7  "<Iin>"
  Bus Selector6/1 -> Mux9/5  "<Iin>"
  Bus Selector8/2 -> Mux9/10  "<Vc>"
  Vmmc_rgt/1 -> Bus Selector/1, Bus Selector1/1
  Bus Selector/1 -> [Varm_T2]
  Bus Selector1/1 -> [AC_brk]  "<brk2>"
  " Switch Identifier1"/1(2sw) -> Simulink-PS Converter6/1
  " Switch Identifier2"/1(2sw) -> Simulink-PS Converter7/1
  " Switch Identifier3"/1(2sw) -> Simulink-PS Converter8/1
  connections:
  Resistor6/RConn1 -- Circuit Breaker1/LConn2 -- Capacitor1/RConn1 -- Inductor Q=50/RConn1
  Inductor Q=50.1/LConn1 -- Current Sensor3/RConn2
  Capacitor/RConn1 -- Electrical Reference1/LConn1 -- Capacitor1/LConn1
  Rs3/RConn1 -- Grounded Neutral (Three-Phase)/LConn1
  Circuit Breaker/RConn1 -- Vdc+(ssc)/RConn1
  SSC_MMC8/LConn1 -- Ls1/RConn1
  Simulink-PS Converter7/RConn1 -- Circuit Breaker/LConn1
  SSC_MMC5/LConn1 -- Ls1/RConn3
  Ls1/LConn1 -- Phase Splitter3/RConn1
  Ls1/LConn2 -- Phase Splitter3/RConn2
  Current Sensor1/RConn1 -- PS-Simulink Converter4/LConn1
  Voltage Sensor5/RConn1 -- PS-Simulink Converter8/LConn1
  Current Sensor4/RConn1 -- PS-Simulink Converter10/LConn1
  Phase Splitter1/RConn3 -- Ls/LConn3
  PS-Simulink Converter3/LConn1 -- Current Sensor3/RConn1
  Voltage Sensor4/RConn1 -- PS-Simulink Converter9/LConn1
  Phase Splitter1/RConn1 -- Ls/LConn1
  Ls1/LConn3 -- Phase Splitter3/RConn3
  SSC_MMC1/LConn2 -- Ls/RConn3
  Vdc-(ssc)/RConn1 -- Circuit Breaker1/RConn1
  Phase Splitter1/RConn2 -- Ls/LConn2
  SSC_MMC3/LConn2 -- Ls/RConn1
  SSC_MMC2/LConn2 -- Ls/RConn2
  SSC_MMC4/LConn1 -- Ls1/RConn2
  Simulink-PS Converter8/RConn1 -- Circuit Breaker1/LConn1
  SSC_MMC3/LConn1 -- Current Sensor4/LConn1
  SSC_MMC5/LConn2 -- Resistor7/RConn1 -- Voltage Sensor5/RConn2 -- Current Sensor1/LConn1 -- SSC_MMC8/LConn2 -- SSC_MMC4/LConn2
  Capacitor/LConn1 -- Circuit Breaker/LConn2 -- Inductor Q=50.1/RConn1 -- Resistor6/LConn1
  SSC_MMC2/LConn1 -- Current Sensor4/RConn2 -- Resistor8/LConn1 -- Current Sensor3/LConn1 -- Voltage Sensor4/LConn1 -- SSC_MMC1/LConn1
  Voltage Sensor5/LConn1 -- Voltage Sensor4/RConn2 -- Resistor8/RConn1 -- Electrical Reference2/LConn1 -- Resistor7/LConn1
  Current Sensor1/RConn2 -- Inductor Q=50/LConn1
  Electrical Reference/LConn1 -- Voltage Source (Three-Phase)/LConn1
  Two-Winding Transformer (Three-Phase)/LConn1 -- Voltage Source (Three-Phase)/RConn1
  PS-Simulink Converter1/LConn1 -- Current and Voltage Sensor (Three-Phase)/RConn1
  Simulink-PS Converter6/RConn1 -- CircuitBreaker/LConn1
  Current and Voltage Sensor (Three-Phase)/RConn2 -- PS-Simulink Converter2/LConn1
  Rs1/RConn1 -- Phase Splitter1/LConn1
  Rs/RConn1 -- Phase Splitter3/LConn1
  Current and Voltage Sensor (Three-Phase)/LConn1 -- CircuitBreaker/RConn1
  Rs/LConn1 -- Rs3/LConn1 -- Current and Voltage Sensor (Three-Phase)/RConn3 -- Rs1/LConn1
  Two-Winding Transformer (Three-Phase)/RConn1 -- Solver Configuration/RConn1 -- CircuitBreaker/LConn2

== system S2/Half-DPL1ph1/Simscape ==
  Electrical Reference1 : fl_lib/Electrical/Electrical Elements/Electrical Reference
  PS-S : nesl_utility/PS-Simulink Converter  PhysicalDomain=network_engine_domain  SubClassName=ps_output  LeftPortType=input  RightPortType=output  PseudoPeriodic=off  Frequencies=[]  VectorFormat=1-D array  Unit=V  AffineConversion=off
  Voltage Sensor : fl_lib/Electrical/Electrical Sensors/Voltage Sensor
  V : PMIOPort  Side=Left
  Out : Outport  VectorParamsAs1DForOutWhenUnconnected=off
  wires:
  PS-S/1 -> Out/1  "voltage"
  connections:
  Electrical Reference1/LConn1 -- Voltage Sensor/RConn2
  V/RConn1 -- Voltage Sensor/LConn1
  PS-S/LConn1 -- Voltage Sensor/RConn1

== system S2/Half-DPL1ph1/Voltage Source ==
  I : Inport
  Controlled Current Source1 : fl_lib/Electrical/Electrical Sources/Controlled Current Source
  Simulink-PS Converter : nesl_utility/Simulink-PS Converter  PhysicalDomain=network_engine_domain  SubClassName=ps_input  LeftPortType=input  RightPortType=output  PseudoPeriodic=off  Frequencies=[]  NoiseDistribution=none  NoiseParameters=[]  Unit=1  AffineConversion=off  FilteringAndDerivatives=zero  SimscapeFilterOrder=1  InputFilterTimeConstant=.001  UdotUserProvided=0
  + : PMIOPort  Side=Right
  - : PMIOPort  Port=2  Side=Right
  wires:
  I/1 -> Simulink-PS Converter/1
  connections:
  Controlled Current Source1/LConn1 -- +/RConn1
  Controlled Current Source1/RConn2 -- -/RConn1
  Controlled Current Source1/RConn1 -- Simulink-PS Converter/RConn1

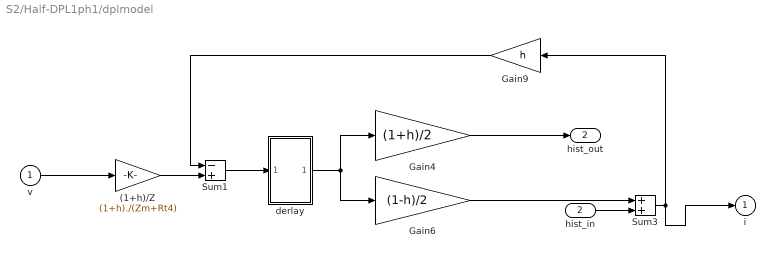
== system S2/Half-DPL1ph1/dplmodel ==
  v : Inport
  hist_in : Inport  Port=2
  (1+h)/Z : Gain  Gain=(1+h)./(Zm+Rt4)  SaturateOnIntegerOverflow=on  OutDataTypeStr=Inherit: Same as input  ParamDataTypeStr=Inherit: Same as input
  Gain4 : Gain  Gain=(1+h)/2  SaturateOnIntegerOverflow=on  OutDataTypeStr=Inherit: Same as input  ParamDataTypeStr=Inherit: Same as input
  Gain6 : Gain  Gain=(1-h)/2  SaturateOnIntegerOverflow=on  OutDataTypeStr=Inherit: Same as input  ParamDataTypeStr=Inherit: Same as input
  Gain9 : Gain  Gain=h  SaturateOnIntegerOverflow=on  OutDataTypeStr=Inherit: Same as input  ParamDataTypeStr=Inherit: Same as input
  Sum1 : Sum  Inputs=-+  InputSameDT=on  SaturateOnIntegerOverflow=on  OutDataTypeStr=Inherit: Same as first input
  Sum3 : Sum  InputSameDT=on  SaturateOnIntegerOverflow=on  OutDataTypeStr=Inherit: Same as first input
  derlay : Subsystem
  i : Outport  InitialOutput=0  VectorParamsAs1DForOutWhenUnconnected=off
  hist_out : Outport  Port=2  VectorParamsAs1DForOutWhenUnconnected=off
  wires:
  Sum1/1 -> derlay/1(In1)
  derlay/1(Out1) -> Gain6/1, Gain4/1
  hist_in/1 -> Sum3/2
  Gain6/1 -> Sum3/1
  (1+h)/Z/1 -> Sum1/2
  Gain9/1 -> Sum1/1
  Gain4/1 -> hist_out/1
  v/1 -> (1+h)/Z/1
  Sum3/1 -> Gain9/1, i/1

== system S2/Half-DPL1ph2/Simscape ==
  Electrical Reference1 : fl_lib/Electrical/Electrical Elements/Electrical Reference
  PS-S : nesl_utility/PS-Simulink Converter  PhysicalDomain=network_engine_domain  SubClassName=ps_output  LeftPortType=input  RightPortType=output  PseudoPeriodic=off  Frequencies=[]  VectorFormat=1-D array  Unit=V  AffineConversion=off
  Voltage Sensor : fl_lib/Electrical/Electrical Sensors/Voltage Sensor
  V : PMIOPort  Side=Left
  Out : Outport  VectorParamsAs1DForOutWhenUnconnected=off
  wires:
  PS-S/1 -> Out/1  "voltage"
  connections:
  PS-S/LConn1 -- Voltage Sensor/RConn1
  V/RConn1 -- Voltage Sensor/LConn1
  Electrical Reference1/LConn1 -- Voltage Sensor/RConn2

== system S2/Half-DPL1ph2/Voltage Source ==
  I : Inport
  Controlled Current Source1 : fl_lib/Electrical/Electrical Sources/Controlled Current Source
  Simulink-PS Converter : nesl_utility/Simulink-PS Converter  PhysicalDomain=network_engine_domain  SubClassName=ps_input  LeftPortType=input  RightPortType=output  PseudoPeriodic=off  Frequencies=[]  NoiseDistribution=none  NoiseParameters=[]  Unit=1  AffineConversion=off  FilteringAndDerivatives=zero  SimscapeFilterOrder=1  InputFilterTimeConstant=.001  UdotUserProvided=0
  + : PMIOPort  Side=Right
  - : PMIOPort  Port=2  Side=Right
  wires:
  I/1 -> Simulink-PS Converter/1
  connections:
  Controlled Current Source1/RConn1 -- Simulink-PS Converter/RConn1
  Controlled Current Source1/RConn2 -- -/RConn1
  Controlled Current Source1/LConn1 -- +/RConn1

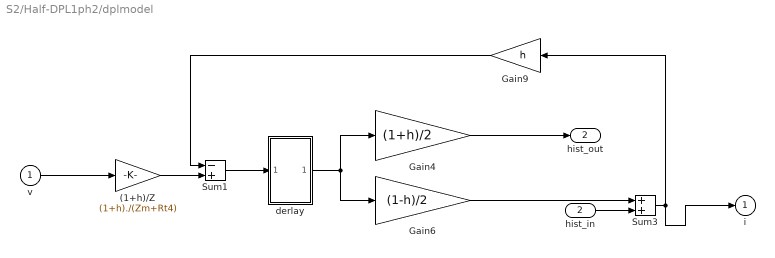
== system S2/Half-DPL1ph2/dplmodel ==
  v : Inport
  hist_in : Inport  Port=2
  (1+h)/Z : Gain  Gain=(1+h)./(Zm+Rt4)  SaturateOnIntegerOverflow=on  OutDataTypeStr=Inherit: Same as input  ParamDataTypeStr=Inherit: Same as input
  Gain4 : Gain  Gain=(1+h)/2  SaturateOnIntegerOverflow=on  OutDataTypeStr=Inherit: Same as input  ParamDataTypeStr=Inherit: Same as input
  Gain6 : Gain  Gain=(1-h)/2  SaturateOnIntegerOverflow=on  OutDataTypeStr=Inherit: Same as input  ParamDataTypeStr=Inherit: Same as input
  Gain9 : Gain  Gain=h  SaturateOnIntegerOverflow=on  OutDataTypeStr=Inherit: Same as input  ParamDataTypeStr=Inherit: Same as input
  Sum1 : Sum  Inputs=-+  InputSameDT=on  SaturateOnIntegerOverflow=on  OutDataTypeStr=Inherit: Same as first input
  Sum3 : Sum  InputSameDT=on  SaturateOnIntegerOverflow=on  OutDataTypeStr=Inherit: Same as first input
  derlay : Subsystem
  i : Outport  InitialOutput=0  VectorParamsAs1DForOutWhenUnconnected=off
  hist_out : Outport  Port=2  VectorParamsAs1DForOutWhenUnconnected=off
  wires:
  Sum3/1 -> i/1, Gain9/1
  v/1 -> (1+h)/Z/1
  Gain4/1 -> hist_out/1
  Gain9/1 -> Sum1/1
  (1+h)/Z/1 -> Sum1/2
  Gain6/1 -> Sum3/1
  hist_in/1 -> Sum3/2
  derlay/1(Out1) -> Gain4/1, Gain6/1
  Sum1/1 -> derlay/1(In1)

== system S2/MMC2/ Switch Identifier1 ==
  in : Inport
  Constant : Constant  Value=rsw
  Switch : Switch  Criteria=u2 > Threshold  Threshold=0.5  SaturateOnIntegerOverflow=off  InputSameDT=off
  inv1 : Subsystem
  2sw : Outport
  wires:
  in/1 -> Switch/3, inv1/1(gate)
  inv1/1(Out1) -> Switch/1
  Switch/1 -> 2sw/1
  Constant/1 -> Switch/2

== system S2/MMC2/ Switch Identifier2 ==
  in : Inport
  Constant : Constant  Value=rsw
  Switch : Switch  Criteria=u2 > Threshold  Threshold=0.5  SaturateOnIntegerOverflow=off  InputSameDT=off
  inv1 : Subsystem
  2sw : Outport
  wires:
  in/1 -> Switch/3, inv1/1(gate)
  inv1/1(Out1) -> Switch/1
  Switch/1 -> 2sw/1
  Constant/1 -> Switch/2

== system S2/MMC2/ Switch Identifier3 ==
  in : Inport
  Constant : Constant  Value=rsw
  Switch : Switch  Criteria=u2 > Threshold  Threshold=0.5  SaturateOnIntegerOverflow=off  InputSameDT=off
  inv1 : Subsystem
  2sw : Outport
  wires:
  in/1 -> Switch/3, inv1/1(gate)
  inv1/1(Out1) -> Switch/1
  Switch/1 -> 2sw/1
  Constant/1 -> Switch/2
